simulink model "ECMO_Device_Project"  (R2020b)
settings: Solver=ode4  StartTime=0.0  StopTime=300  FixedStep=Tsamp  RelTol=1e-3
model workspace (MATLAB code in the model file):
  | %%%%%%%%%%%%%%%%%%%%%%%%%%%%%%%%%%%%%%%%%%%%%%%%%%%
  | %%%%%%%%%%%%% Term Project Parameters %%%%%%%%%%%%%
  | %%%%%%%%%%%%%%%%%%%%%%%%%%%%%%%%%%%%%%%%%%%%%%%%%%%
  | 
  | %% Physiological/Environmental Parameters
  | Tsamp = 1e-3;      % s
  | FIO2 = 50/100;  % (%) (Change this to 50% when ECMO is initiated)
  | FICO2 = 0.0/100;   % (%)
  | Patm = 760.0;      % mmHg
  | Pws = 47.0;        % mmHg
  | shunt = 36.5/100;  % (%)
  | 
  | %% Parameters of the Lung Mechanics
  | Clung = 0.062;     % l/cmH2O
  | Rtube = 3.76;      % cmH2O.s.l^-1
  | Rlung = 1.4013;    % cmH2O.s.l^-1
  | VL0 = 3.40;        % l
  | VReference = 0.2;  % l  (Change this to 0.2 l when ECMO is initiated)
  | 
  | %% Parameters of the Dead-Space
  | VD = 0.15;         % l
  | PdO2_IC = 60.0;    % mmHg
  | PdCO2_IC = 53.0;   % mmHg
  | 
  | %% Parameters of the Alveolar Gas Exchange
  | PAO2_IC = 57.0;    % mmHg
  | PACO2_IC = 55.0;   % mmHg
  | CaO2_IC = 0.184;   % ml/ml
  | CaCO2_IC = 0.565;  % ml/ml
  | Tau_TL = 10.0;     % s
  | kEff = 0.55;
  | 
  | %% Parameters of the Blood Dissociation Curves
  | CsatO2 = 0.2128;   % ml/ml
  | alpha1 = 0.03198;  % mmHg^-1
  | beta1 = 0.008275;  % mmHg^-1
  | K1 = 15.0;         % mmHg
  | h1 = 0.3836;
  | 
  | CsatCO2 = 1.9488;  % ml/ml
  | alpha2 = 0.05591;  % mmHg^-1
  | beta2 = 0.03255;   % mmHg^-1
  | K2 = 194.4;        % mmHg
  | h2 = 1.819;
  | 
  | %% Parameters of the Tissue Gas Exchange
  | VTO2 = 7700;       % ml
  | VTCO2 = 6000;      % ml
  | MRO2 = 3.80;       % ml/s
  | MRCO2 = 3.30;      % ml/s
  | CvO2_IC = 0.134;   % ml/ml
  | CvCO2_IC = 0.602;  % ml/ml
  | Tau_LT = 18.0;     % s
  | 
  | %% ECMO Pump Parameters
  | R = 10.0;     % ohm
  | L = 10.0;     % mH
  | kem = 0.192;  % V/(rd/s)
  | JL = 8e-4;    % kg.m^2
  | Ng = 0.5;
  | 
  | %% ECMO Oxygenator Parameters
  | VEO2 = 1.5;       % l
  | VECO2 = 1.5;      % l
  | PEO2_IC = 200.0;  % mmHg
  | PECO2_IC = 40.0;  % mmHg
  | 
  | FIEO2 = 100/100;   % (%)
  |  % (Change this to initiate ECMO)
libraries: fl_lib x19, nesl_utility x7, pid_lib x4
(part 2 of 2)

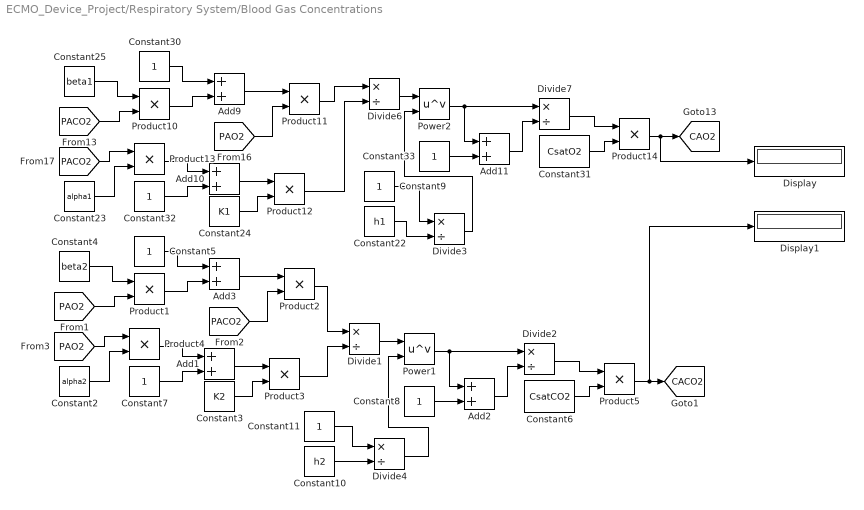
== system ECMO_Device_Project/Respiratory System/Blood Gas Concentrations  ==
  Add{1..3,9..11} (6 alike) : Sum
  Constant10 : Constant  Value=h2  SampleTime=Tsamp
  Constant{5,7..9,11,30,32..33} (8 alike) : Constant  SampleTime=Tsamp
  Constant2 : Constant  Value=alpha2  SampleTime=Tsamp
  Constant22 : Constant  Value=h1  SampleTime=Tsamp
  Constant23 : Constant  Value=alpha1  SampleTime=Tsamp
  Constant24 : Constant  Value=K1  SampleTime=Tsamp
  Constant25 : Constant  Value=beta1  SampleTime=Tsamp
  Constant3 : Constant  Value=K2  SampleTime=Tsamp
  Constant31 : Constant  Value=CsatO2  SampleTime=Tsamp
  Constant4 : Constant  Value=beta2  SampleTime=Tsamp
  Constant6 : Constant  Value=CsatCO2  SampleTime=Tsamp
  Display : Display
  Display1 : Display
  Divide{1..4,6..7} (6 alike) : Product  Inputs=*/
  Power1 : Math  Operator=pow  SaturateOnIntegerOverflow=on
  Power2 : Math  Operator=pow  SaturateOnIntegerOverflow=on
  Product{1..5,10..14} (10 alike) : Product
  tag scope: CACO2=global, CAO2=global
  wires:
  Constant24/1 -> Product12/2
  Power2/1 -> Add11/1, Divide7/1
  Add10/1 -> Product12/1
  Product10/1 -> Add9/2
  Divide7/1 -> Product14/1
  Product12/1 -> Divide6/2
  Product13/1 -> Add10/1
  Constant33/1 -> Add11/2
  Constant23/1 -> Product13/2
  Constant30/1 -> Add9/1
  Add9/1 -> Product11/1
  Constant32/1 -> Add10/2
  Product14/1 -> Display/1, [CAO2]
  Constant25/1 -> Product10/1
  [PAO2] -> Product11/2
  Add11/1 -> Divide7/2
  Product11/1 -> Divide6/1
  Constant31/1 -> Product14/2
  [PACO2] -> Product10/2
  [PACO2] -> Product13/1
  Add3/1 -> Product2/1
  Constant2/1 -> Product4/2
  Constant5/1 -> Add3/1
  Constant8/1 -> Add2/2
  Divide2/1 -> Product5/1
  Add1/1 -> Product3/1
  Power1/1 -> Add2/1, Divide2/1
  Product1/1 -> Add3/2
  Product3/1 -> Divide1/2
  Constant3/1 -> Product3/2
  Product4/1 -> Add1/1
  Add2/1 -> Divide2/2
  Product5/1 -> Display1/1, [CACO2]
  Product2/1 -> Divide1/1
  [PAO2] -> Product4/1
  Constant7/1 -> Add1/2
  [PACO2] -> Product2/2
  Constant4/1 -> Product1/1
  [PAO2] -> Product1/2
  Constant6/1 -> Product5/2
  Divide1/1 -> Power1/1
  Divide4/1 -> Power1/2
  Divide6/1 -> Power2/1
  Constant22/1 -> Divide3/2
  Divide3/1 -> Power2/2
  Constant9/1 -> Divide3/1
  Constant11/1 -> Divide4/1
  Constant10/1 -> Divide4/2

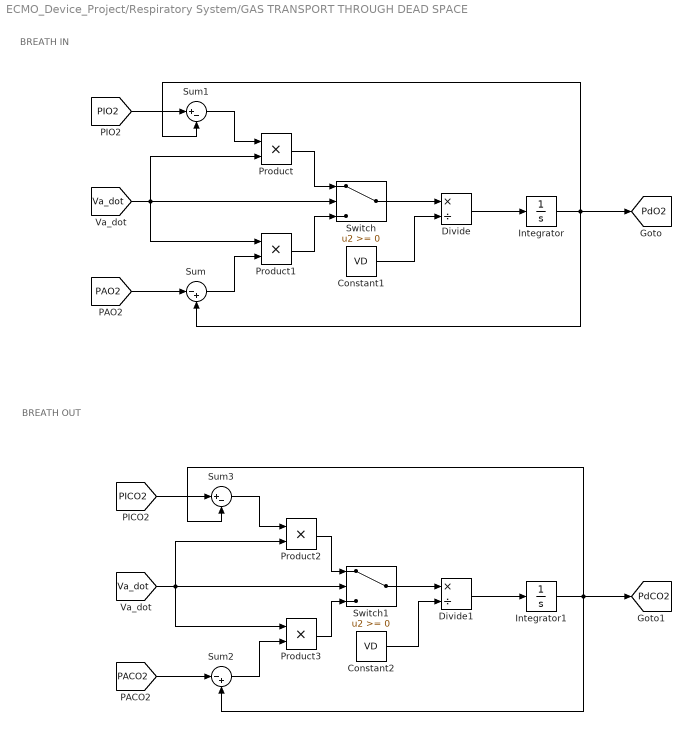
== system ECMO_Device_Project/Respiratory System/GAS TRANSPORT THROUGH DEAD SPACE ==
  note: BREATH IN
  note: BREATH OUT
  Constant1 : Constant  Value=VD  SampleTime=Tsamp
  Constant2 : Constant  Value=VD  SampleTime=Tsamp
  Divide : Product  Inputs=*/
  Divide1 : Product  Inputs=*/
  Integrator : Integrator  InitialCondition=PdO2_IC
  Integrator1 : Integrator  InitialCondition=PdCO2_IC
  Product{,1..3} (4 alike) : Product
  Sum : Sum  Inputs=|-+
  Sum1 : Sum  Inputs=|+-
  Sum2 : Sum  Inputs=|-+
  Sum3 : Sum  Inputs=|+-
  Switch : Switch
  Switch1 : Switch
  tag scope: PdCO2=global, PdO2=global
  wires:
  Integrator1/1 -> [PdCO2], Sum2/2, Sum3/2
  Product1/1 -> Switch/3
  [Va_dot] -> Switch/2, Product1/1, Product/2
  [PIO2] -> Sum1/1
  Integrator/1 -> [PdO2], Sum/2, Sum1/2
  Sum1/1 -> Product/1
  Sum/1 -> Product1/2
  Switch/1 -> Divide/1
  [Va_dot] -> Switch1/2, Product3/1, Product2/2
  [PICO2] -> Sum3/1
  Product/1 -> Switch/1
  Constant1/1 -> Divide/2
  Divide1/1 -> Integrator1/1
  Constant2/1 -> Divide1/2
  Product2/1 -> Switch1/1
  Divide/1 -> Integrator/1
  [PACO2] -> Sum2/1
  Sum2/1 -> Product3/2
  Switch1/1 -> Divide1/1
  Product3/1 -> Switch1/3
  Sum3/1 -> Product2/1
  [PAO2] -> Sum/1

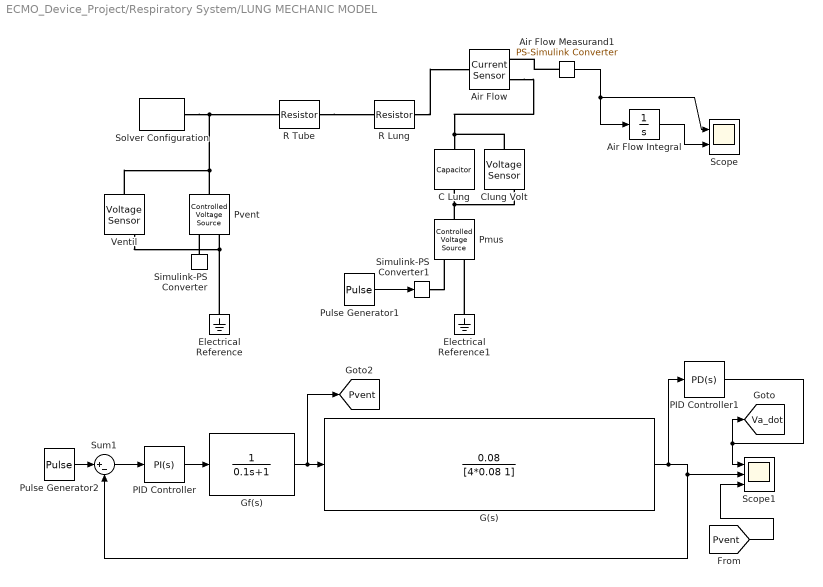
== system ECMO_Device_Project/Respiratory System/LUNG MECHANIC MODEL ==
  Air Flow : fl_lib/Electrical/Electrical Sensors/Current Sensor
  Air Flow Measurand1 : nesl_utility/PS-Simulink Converter  PhysicalDomain=network_engine_domain  SubClassName=ps_output  LeftPortType=input  RightPortType=output  PseudoPeriodic=off  Frequencies=[]  Unit=inherit  AffineConversion=off
  Air Flow Integral : Integrator  InitialCondition=VReference
  C Lung : fl_lib/Electrical/Electrical Elements/Capacitor  c=Clung F  r=Clung Ohm  g=0 1/Ohm  i_specify=off  i_priority=None  i=0 A  i_nominal_specify=off  i_nominal_unit=A  i_nominal_value=1  v_specify=off  v_priority=None  v=0 V  v_nominal_specify=off  v_nominal_unit=V  v_nominal_value=1  vc_specify=off  vc_priority=High  vc=0 V  vc_nominal_specify=off  vc_nominal_unit=V  vc_nominal_value=1
  Clung Volt : fl_lib/Electrical/Electrical Sensors/Voltage Sensor
  Electrical Reference : fl_lib/Electrical/Electrical Elements/Electrical Reference
  Electrical Reference1 : fl_lib/Electrical/Electrical Elements/Electrical Reference
  "G(s) " : TransferFcn  Numerator=[0.08]  Denominator=[4*0.08 1]
  "Gf(s) " : TransferFcn  Denominator=[0.1 1]
  PID Controller : pid_lib/PID Controller  Controller=PI  Form=Parallel  TimeDomain=Continuous-time  UseExternalTs=off  SampleTime=-1  IntegratorMethod=Forward Euler  FilterMethod=Forward Euler  ControllerParametersSource=internal  P=11.56  I=3.125*11.56  D=0  UseFilter=on  N=100  TunerSelectOption=Transfer Function Based (PID Tuner App)  InitialConditionSource=internal  InitialConditionForIntegrator=0  InitialConditionForFilter=0  DifferentiatorICPrevScaledInput=0  ExternalReset=none  TrackingMode=off  Kt=1  LimitOutput=on  SatLimitsSource=internal  UpperSaturationLimit=inf  LowerSaturationLimit=0  LinearizeAsGain=on  AntiWindupMode=back-calculation  Kb=1  POutMin=[]  POutMax=[]  IOutMin=[]  IOutMax=[]  DOutMin=[]  DOutMax=[]  NOutMin=[]  NOutMax=[]  SumOutMin=[]  SumOutMax=[]  SaturationOutMin=[]  SaturationOutMax=[]  PParamMin=[]  PParamMax=[]  IParamMin=[]  IParamMax=[]  DParamMin=[]  DParamMax=[]  NParamMin=[]  NParamMax=[]  KbParamMin=[]  KbParamMax=[]  KtParamMin=[]  KtParamMax=[]  KbOutMin=[]  KbOutMax=[]  KtOutMin=[]  KtOutMax=[]  IntegratorOutMin=[]  IntegratorOutMax=[]  FilterOutMin=[]  FilterOutMax=[]  SumI1OutMin=[]  SumI1OutMax=[]  SumI2OutMin=[]  SumI2OutMax=[]  SumI3OutMin=[]  SumI3OutMax=[]  SumI4OutMin=[]  SumI4OutMax=[]  SumDOutMin=[]  SumDOutMax=[]  DifferentiatorOutMin=[]  DifferentiatorOutMax=[]  FilterDiffOutCoefMin=[]  FilterDiffOutCoefMax=[]  ReciprocalOutMin=[]  ReciprocalOutMax=[]  SumDenOutMin=[]  SumDenOutMax=[]  SumNumOutMin=[]  SumNumOutMax=[]  DivideOutMin=[]  DivideOutMax=[]  UdiffTsProdOutMin=[]  UdiffTsProdOutMax=[]  NTsProdOutMin=[]  NTsProdOutMax=[]  UintegralTsProdOutMin=[]  UintegralTsProdOutMax=[]  UngainTsProdOutMin=[]  UngainTsProdOutMax=[]  IntegratorContinuousStateAttributes=''  IntegratorStateMustResolveToSignalObject=off  IntegratorRTWStateStorageClass=Auto  FilterContinuousStateAttributes=''  FilterStateMustResolveToSignalObject=off  FilterRTWStateStorageClass=Auto  ParallelPVariant=InternalParameters  IdealPVariant=Disabled  IVariant=InternalParameters  DVariant=Disabled  IntegratorVariant=Continuous  SatVariant=Enabled  AWVariant=BackCalculation  PCopyVariant=Disabled  TRVariant=Disabled  FdbkBlocksVariant=Forward  IdealPFdbkVariant=Disabled  SatFdbkVariant=Disabled  DerivativeFilterVariant=Disabled  NVariant=Disabled  NCopyVariant=Disabled_SignalSpec  FilterICVariant=Disabled  IntegratorICVariant=InternalICs  ExternalResetVariant=Disabled  TRSumVariant=Passthrough  SumFdbkVariant=Disabled  SumVariant=Sum_PI  TsampFilterVariant=InternalTs  TsampNgainVariant=Passthrough  TsampIntegralVariant=Passthrough  ExternalSaturationOutDataTypeStr=Inherit: Same as second input
  PID Controller1 : pid_lib/PID Controller  Controller=PD  Form=Parallel  TimeDomain=Continuous-time  UseExternalTs=off  SampleTime=-1  IntegratorMethod=Forward Euler  FilterMethod=Forward Euler  ControllerParametersSource=internal  P=0  I=36.125  D=1  UseFilter=on  N=100  TunerSelectOption=Transfer Function Based (PID Tuner App)  InitialConditionSource=internal  InitialConditionForIntegrator=0  InitialConditionForFilter=0  DifferentiatorICPrevScaledInput=0  ExternalReset=none  TrackingMode=off  Kt=1  LimitOutput=on  SatLimitsSource=internal  UpperSaturationLimit=inf  LowerSaturationLimit=-inf  LinearizeAsGain=on  AntiWindupMode=back-calculation  Kb=1  POutMin=[]  POutMax=[]  IOutMin=[]  IOutMax=[]  DOutMin=[]  DOutMax=[]  NOutMin=[]  NOutMax=[]  SumOutMin=[]  SumOutMax=[]  SaturationOutMin=[]  SaturationOutMax=[]  PParamMin=[]  PParamMax=[]  IParamMin=[]  IParamMax=[]  DParamMin=[]  DParamMax=[]  NParamMin=[]  NParamMax=[]  KbParamMin=[]  KbParamMax=[]  KtParamMin=[]  KtParamMax=[]  KbOutMin=[]  KbOutMax=[]  KtOutMin=[]  KtOutMax=[]  IntegratorOutMin=[]  IntegratorOutMax=[]  FilterOutMin=[]  FilterOutMax=[]  SumI1OutMin=[]  SumI1OutMax=[]  SumI2OutMin=[]  SumI2OutMax=[]  SumI3OutMin=[]  SumI3OutMax=[]  SumI4OutMin=[]  SumI4OutMax=[]  SumDOutMin=[]  SumDOutMax=[]  DifferentiatorOutMin=[]  DifferentiatorOutMax=[]  FilterDiffOutCoefMin=[]  FilterDiffOutCoefMax=[]  ReciprocalOutMin=[]  ReciprocalOutMax=[]  SumDenOutMin=[]  SumDenOutMax=[]  SumNumOutMin=[]  SumNumOutMax=[]  DivideOutMin=[]  DivideOutMax=[]  UdiffTsProdOutMin=[]  UdiffTsProdOutMax=[]  NTsProdOutMin=[]  NTsProdOutMax=[]  UintegralTsProdOutMin=[]  UintegralTsProdOutMax=[]  UngainTsProdOutMin=[]  UngainTsProdOutMax=[]  IntegratorContinuousStateAttributes=''  IntegratorStateMustResolveToSignalObject=off  IntegratorRTWStateStorageClass=Auto  FilterContinuousStateAttributes=''  FilterStateMustResolveToSignalObject=off  FilterRTWStateStorageClass=Auto  ParallelPVariant=InternalParameters  IdealPVariant=Disabled  IVariant=Disabled  DVariant=InternalParameters  IntegratorVariant=Disabled  SatVariant=Enabled  AWVariant=Disabled  PCopyVariant=Disabled  TRVariant=Disabled  FdbkBlocksVariant=Forward  IdealPFdbkVariant=Disabled  SatFdbkVariant=Disabled  DerivativeFilterVariant=ContFilter  NVariant=InternalParameters  NCopyVariant=Disabled  FilterICVariant=InternalICsFilter  IntegratorICVariant=Disabled  ExternalResetVariant=Disabled  TRSumVariant=Passthrough  SumFdbkVariant=Disabled  SumVariant=Sum_PD  TsampFilterVariant=InternalTs  TsampNgainVariant=Passthrough  TsampIntegralVariant=Disabled_SignalSpec  ExternalSaturationOutDataTypeStr=Inherit: Same as second input
  Pmus : fl_lib/Electrical/Electrical Sources/Controlled Voltage Source
  Pulse Generator1 : DiscretePulseGenerator  PulseType=Time based  Amplitude=0  Period=5  PulseWidth=35
  Pulse Generator2 : DiscretePulseGenerator  PulseType=Time based  Amplitude=VReference  Period=5  PulseWidth=35
  Pvent : fl_lib/Electrical/Electrical Sources/Controlled Voltage Source
  R Lung : fl_lib/Electrical/Electrical Elements/Resistor  R=Rlung Ohm  i_specify=off  i_priority=None  i=0 A  i_nominal_specify=off  i_nominal_unit=A  i_nominal_value=1  v_specify=off  v_priority=None  v=0 V  v_nominal_specify=off  v_nominal_unit=V  v_nominal_value=1
  R Tube : fl_lib/Electrical/Electrical Elements/Resistor  R=Rtube Ohm  i_specify=off  i_priority=None  i=0 A  i_nominal_specify=off  i_nominal_unit=A  i_nominal_value=1  v_specify=off  v_priority=None  v=0 V  v_nominal_specify=off  v_nominal_unit=V  v_nominal_value=1
  Scope : Scope  NumInputPorts=2
  Scope1 : Scope  NumInputPorts=3
  Simulink-PS Converter : nesl_utility/Simulink-PS Converter  PhysicalDomain=network_engine_domain  SubClassName=ps_input  LeftPortType=input  RightPortType=output  PseudoPeriodic=off  Frequencies=[]  NoiseDistribution=none  NoiseParameters=[]  Unit=1  AffineConversion=off  FilteringAndDerivatives=provide  SimscapeFilterOrder=1  InputFilterTimeConstant=0.001  UdotUserProvided=0
  Simulink-PS Converter1 : nesl_utility/Simulink-PS Converter  PhysicalDomain=network_engine_domain  SubClassName=ps_input  LeftPortType=input  RightPortType=output  PseudoPeriodic=off  Frequencies=[]  NoiseDistribution=none  NoiseParameters=[]  Unit=1  AffineConversion=off  FilteringAndDerivatives=provide  SimscapeFilterOrder=1  InputFilterTimeConstant=0.001  UdotUserProvided=0
  Solver Configuration : nesl_utility/Solver Configuration  PhysicalDomain=network_engine_domain  SubClassName=solver  LeftPortType=input  RightPortType=generic  Tones=[]  Harmonics=[]  SimulateNoise=off  Profile=off  UseLocalSampling=off  EnableSwitchedLinearOptims=on  FrequencyDomain=off  UseCCode=off  RelTol=0.001  AbsTol=1e-06  MinStep=1e-09  ToWorkspace=off  RevertToSquareIcSolve=off  NumHomotopyIterations=100  PhasorMode=off  PhasorModeNumHarmonics=1  DoDC=off  ResidualTolerance=1e-09  UseLocalSolver=off  LocalSolverChoice=NE_BACKWARD_EULER_ADVANCER  LocalSolverSampleTime=0.001  DoFixedCost=off  MaxNonlinIter=3  MaxModeIter=2  ComputeImpulses=off  ImpulseIterations=2  LinearAlgebra=auto  EquationFormulation=NE_TIME_EF  DelaysMemoryBudget=1024  AutomaticFiltering=on  FilteringTimeConstant=0.001  PartitionStorageMethod=AS_NEEDED  PartitionMemoryBudget=1024  PartitionMethod=ROBUST
  Sum1 : Sum  Inputs=|+-
  Ventil : fl_lib/Electrical/Electrical Sensors/Voltage Sensor
  tag scope: Pvent=global, Va_dot=global
  wires:
  Pulse Generator1/1 -> Simulink-PS Converter1/1
  Air Flow Measurand1/1 -> Air Flow Integral/1, Scope/1
  Air Flow Integral/1 -> Scope/2
  PID Controller/1 -> "Gf(s) "/1
  Pulse Generator2/1 -> Sum1/1
  Sum1/1 -> PID Controller/1
  "Gf(s) "/1 -> [Pvent], "G(s) "/1
  "G(s) "/1 -> PID Controller1/1, Sum1/2, Scope1/2
  PID Controller1/1 -> [Va_dot], Scope1/1
  [Pvent] -> Scope1/3
  connections:
  R Tube/RConn1 -- R Lung/LConn1
  Air Flow Measurand1/LConn1 -- Air Flow/RConn1
  Clung Volt/LConn1 -- Air Flow/RConn2 -- C Lung/LConn1
  Simulink-PS Converter/RConn1 -- Pvent/RConn1
  R Lung/RConn1 -- Air Flow/LConn1
  Electrical Reference1/LConn1 -- Pmus/RConn2
  Pmus/LConn1 -- Clung Volt/RConn2 -- C Lung/RConn1
  Electrical Reference/LConn1 -- Ventil/RConn2 -- Pvent/RConn2
  Pvent/LConn1 -- Ventil/LConn1 -- Solver Configuration/RConn1 -- R Tube/LConn1
  Simulink-PS Converter1/RConn1 -- Pmus/RConn1

== matlab function ECMO_Device_Project/CARDIO PUMP MODEL/MATLAB Function4 ==
  data: t input; y output
function y = fcn(t)
y = (abs((sin(pi*t/0.19)))^2)*670+1;

== matlab function ECMO_Device_Project/CARDIO PUMP MODEL/MOD2 ==
  data: t input; y output
function y = fcn(t)
    period=mod(t,0.84);
y = period;

== matlab function ECMO_Device_Project/CARDIO PUMP MODEL/MATLAB Function1 ==
  data: t input; y output
function y = fcn(t)
y = (abs((sin(pi*t/0.25)))^1.55)*460+1;
